simulink model "ofdm_13"  (Simulink 7.4)
settings: Solver=FixedStepDiscrete  SolverMode=SingleTasking  StartTime=0.0  StopTime=inf  MaxStep=1/(100*40e6)  RelTol=1e-3
PreLoadFcn:
  | Fsymbol              = .5e6;         % Symbol rate
  | D=8;  % decimation / interpolation
  | Bits_per_Symbol = 2;
  | Fbit  = Bits_per_Symbol*Fsymbol;
  | 
  | FFT_Size  = 64;
  | Cyclic        = 16;
  | Pilots         = 16;
  | Pilot_Level = 8;
  | Zero_Pad  = 3;
  | QAM_Level = 6;
  | 
  | OFDM_Frame =  FFT_Size+Cyclic;
  | Symbols_per_Frame = FFT_Size-Pilots-Zero_Pad;
  | 
  | Bits_per_Frame = Bits_per_Symbol*Symbols_per_Frame;
  | 
  | F_nco = Fsymbol*D*OFDM_Frame/(Symbols_per_Frame);
  | nco_nominal=2/D;
  | 
  | 
  | Fdelay = 8;  % rrc filter delay
  | Alpha = .25;  % excess BW
  | rrc_coef=rcosine(1,D,'fir/sqrt',Alpha,Fdelay);
  | rrc_coef=rrc_coef/sum(rrc_coef);
  | 
  | 
  | % coefficents for Farrow filter
  | b3 = [1/6 -1/2  1/2 -1/6];
  | b2 = [1/2 -1    1/2  0];
  | b1 = [1/3  1/2 -1    1/6];
  | b0 = [0    1    0    0];
StartFcn:
  | tic
StopFcn:
  | trun=toc
values from neighbouring files (symbols this model uses):
  Fs = 1    [16 qam.m]    (also in G.m = input('Enter sampling frequency='))
  j = imread('lena.jpg')    [ansk3.m]    (also in cosine_filter.m = 2; imag1.m)
  N = [N1;N2;N1_;N2_]    [FFT_OFDM_MIMO.m]    (also in MRCplot.m = 1000000; SDplot.m = 1000000; ansk2.m = 10; ansk3.m = 10)
undefined symbols (not defined in the file or in its folder): dBW, dfilt, Hz, magnitude, sided, Ts, Two
libraries: simulink x25, dspobslib x22, dspsigops x13, dspbuff3 x5, dspsnks4 x4, dspxfrm3 x4, dspstat3 x4, commsink2 x3, commchan3 x2, dsparch4 x2, commrandsrc2 x2, commdigbbndam3 x2
(part 2 of 2)

== system ofdm_13/OFDM Transmitter with Variable Symbol Timing and Carrier Frequency Error/Discrete-Time NCO ==
  note: initial condx=Ph
  note: VCO Sensitivity
  note: Center Freq
  note: Phase Accumulator
      | Modulus
  note: Amplitude
  in_1 : Inport  OutDataType=sfix(16)  OutScaling=2^0
  Discrete Constant1 : dspobslib/DSP Constant  SystemSampleTime=-1  Value=Fc*pi2*ts  SampleMode=Discrete  discreteOutput=Sample-based (interpret vectors as 1-D)  continuousOutput=Sample-based  sampTime=ts  framePeriod=ts  dataType=Inherit via back propagation  isSigned=on  wordLen=16  udDataType=sfix(16)  fracBitsMode=Best precision  numFracBits=15  InterpretAs1D=on  Ts=ts  FramebasedOutput=off
      settings: additionalParams=on
  Discrete Constant2 : dspobslib/DSP Constant  SystemSampleTime=-1  Value=pi2  SampleMode=Discrete  discreteOutput=Sample-based (interpret vectors as 1-D)  continuousOutput=Sample-based  sampTime=ts  framePeriod=ts  dataType=Inherit via back propagation  isSigned=on  wordLen=16  udDataType=sfix(16)  fracBitsMode=Best precision  numFracBits=15  InterpretAs1D=on  Ts=ts  FramebasedOutput=off
      settings: additionalParams=on
  Math Function : Math  Operator=mod  OutDataType=sfix(16)  OutScaling=2^0  SaturateOnIntegerOverflow=on
  Real-Imag to Complex : RealImagToComplex
  Sensitivity : Gain  Gain=Kc*pi2*ts  ParameterDataType=sfix(16)  ParameterScaling=2^0  OutDataType=sfix(16)  OutScaling=2^0  SaturateOnIntegerOverflow=on  OutDataTypeStr=Inherit: Same as input  ParamDataTypeStr=Inherit: Same as input
  Sensitivity2 : Gain  Gain=Ac  ParameterDataType=sfix(16)  ParameterScaling=2^0  OutDataType=sfix(16)  OutScaling=2^0  SaturateOnIntegerOverflow=on  OutDataTypeStr=Inherit: Same as input  ParamDataTypeStr=Inherit: Same as input
  Sum1 : Sum  Inputs=+++  OutDataType=sfix(16)  OutScaling=2^0  SaturateOnIntegerOverflow=on  InputSameDT=on  OutDataTypeStr=Inherit: Same as first input
  Trigonometric Function : Trigonometry  Operator=cos
  Trigonometric Function1 : Trigonometry
  Unit Delay : UnitDelay  X0=Ph  SampleTime=ts
  out_1 : Outport  OutDataType=sfix(16)  OutScaling=2^0  InitialOutput=0
  wires:
  Real-Imag to Complex/1 -> Sensitivity2/1
  Trigonometric Function1/1 -> Real-Imag to Complex/2
  Discrete Constant2/1 -> Math Function/2
  Sum1/1 -> Math Function/1
  Math Function/1 -> Unit Delay/1
  in_1/1 -> Sensitivity/1
  Sensitivity/1 -> Sum1/1
  Unit Delay/1 -> Trigonometric Function/1, Trigonometric Function1/1, Sum1/3
  Trigonometric Function/1 -> Real-Imag to Complex/1
  Sensitivity2/1 -> out_1/1
  Discrete Constant1/1 -> Sum1/2

== system ofdm_13/OFDM Transmitter with Variable Symbol Timing and Carrier Frequency Error/Farrow Variable Delay ==
  Xin : Inport  OutDataType=sfix(16)  OutScaling=2^0
  Mu : Inport  Port=2  OutDataType=sfix(16)  OutScaling=2^0
  Filter State : Subsystem
  MADS : Subsystem
  Yout : Outport  OutDataType=sfix(16)  OutScaling=2^0
  wires:
  Filter State/1(Out1) -> MADS/1(In1)
  Xin/1 -> Filter State/1(In1)
  Mu/1 -> MADS/2(mu)
  MADS/1(Yout) -> Yout/1

== system ofdm_13/OFDM Transmitter with Variable Symbol Timing and Carrier Frequency Error/OFDM Symbol Gen ==
  note: Output Samples Serially
  note: Note: Ouptut is SET TO ZERO
      | when not enabled.
      | This effecitvly inserts ZEROS in the stream
      | for proper interpolation.
  Enable : EnablePort
  Divide by  OFDM_Frame length : Subsystem  TreatAsAtomicUnit=on  mask(Pulse Divider){div=OFDM_Frame, ph=0}
      mask prompts: div "Modulo:"; ph "Initial Phase Delay (cycles):"
  OFDM Generator : Subsystem
  Selector : Selector  InputPortWidth=80  IndexOptions=Index vector (port)  Indices=[1 3]  OutputSizes=1
  Serial Samples Out : Outport  OutDataType=sfix(16)  OutScaling=2^0  OutputWhenDisabled=reset  InitialOutput=0+j*eps
  wires:
  OFDM Generator/1(Out1) -> Selector/1
  Divide by  OFDM_Frame length/1(Enable) -> OFDM Generator/Enable
  Selector/1 -> Serial Samples Out/1
  Divide by  OFDM_Frame length/2(Count) -> Selector/2

== system ofdm_13/OFDM Transmitter with Variable Symbol Timing and Carrier Frequency Error/Timing Control Unit1 ==
  note: Numerically Controlled Oscillator
  Control In : Inport  OutDataType=sfix(16)  OutScaling=2^0
  Delay2 : dspsigops/Delay  dly_unit=Samples  delay=1  ic_detail=on  dif_ic_for_ch=off  dif_ic_for_dly=off  ic=0  reset_popup=None
  Discrete Constant1 : dspobslib/DSP Constant  SystemSampleTime=-1  Value=1  SampleMode=Discrete  discreteOutput=Sample-based (interpret vectors as 1-D)  continuousOutput=Sample-based  sampTime=inf  framePeriod=inf  dataType=Inherit via back propagation  isSigned=on  wordLen=16  udDataType=sfix(16)  fracBitsMode=Best precision  numFracBits=15  InterpretAs1D=on  Ts=inf  FramebasedOutput=off
      settings: additionalParams=on
  Math Function : Math  Operator=mod  OutDataType=sfix(16)  OutScaling=2^0  SaturateOnIntegerOverflow=on
  Relational Operator1 : RelationalOperator  Operator=~=  LogicOutDataTypeMode=boolean  LogicDataType=double(64)  OutDataTypeStr=boolean
  S&H 1 : Subsystem  TreatAsAtomicUnit=on
  Scaling1 : Subsystem
  Sum2 : Sum  Inputs=-+  OutDataType=sfix(16)  OutScaling=2^0  SaturateOnIntegerOverflow=on  InputSameDT=on  OutDataTypeStr=Inherit: Same as first input
  Clock Out : Outport  OutDataType=sfix(16)  OutScaling=2^0
  Delay Control : Outport  Port=2  OutDataType=sfix(16)  OutScaling=2^0
  wires:
  Scaling1/1(Out1) -> Delay Control/1
  S&H 1/1(Out1) -> Scaling1/1(In1)
  Delay2/1 -> Math Function/1, Relational Operator1/1
  Discrete Constant1/1 -> Math Function/2
  Sum2/1 -> Delay2/1
  Math Function/1 -> Relational Operator1/2, S&H 1/1(In1), Sum2/2
  Relational Operator1/1 -> Clock Out/1, S&H 1/Enable
  Control In/1 -> Sum2/1, Scaling1/2(In2)

== system ofdm_13/Serial to Parallel and Frame Offset Est/Cyclic Prefix Correlation for Frame  Boundary Estimation ==
  note: http://citeseer.ist.psu.edu/cache/papers/cs/27222/http:zSzzSzwww.sm.luth.sezSzcseezSzspzSzresearchzSzconferencezSzbsb96c.pdf/on-synchronization-in-ofdm.pdf
  note: Google " On Synchronization in OFDM Systems Using the Cyclic Prefix "
  Strobe : Inport
  Serial : Inport  Port=2
  Estimators : Subsystem
  Find max : Subsystem
  Terminator : Terminator
  buffer one frame worth : dspbuff3/Delay Line  siz=OFDM_Frame  ic=0  directfeed=on  enable_output=off  hold_output=off
  Offset in Samples : Outport
  wires:
  Estimators/1(Delay Est Data) -> buffer one frame worth/1
  buffer one frame worth/1 -> Find max/1(In1)
  Estimators/2(Freq Error Est) -> Terminator/1
  Strobe/1 -> Find max/Enable
  Serial/1 -> Estimators/1(In1)
  Find max/1(Frame Offset Est) -> Offset in Samples/1

== system ofdm_13/Timing Control Unit/Compute % Error from Nominal value ==
  In : Inport
  Add : Sum  Inputs=+-  OutDataType=sfix(16)  OutScaling=2^-10
  Discrete Constant3 : dspobslib/DSP Constant  SystemSampleTime=-1  Value=1  SampleMode=Discrete  discreteOutput=Sample-based (interpret vectors as 1-D)  continuousOutput=Sample-based  sampTime=2/F_nco  framePeriod=2/F_nco  dataType=Inherit via back propagation  isSigned=on  wordLen=16  udDataType=sfix(16)  fracBitsMode=Best precision  numFracBits=15  InterpretAs1D=on  Ts=2/F_nco  FramebasedOutput=off
      settings: additionalParams=on
  Gain : Gain  Gain=1/nco_nominal  ParameterDataType=sfix(16)  ParameterScaling=2^0  OutDataType=sfix(16)  OutScaling=2^0
  Gain1 : Gain  Gain=100  ParameterDataType=sfix(16)  ParameterScaling=2^0  OutDataType=sfix(16)  OutScaling=2^0
  Out : Outport
  wires:
  Gain1/1 -> Out/1
  In/1 -> Gain/1
  Discrete Constant3/1 -> Add/2
  Add/1 -> Gain1/1
  Gain/1 -> Add/1

== system ofdm_13/Timing Control Unit/Sample & Scale ==
  In1 : Inport  OutDataType=sfix(16)  OutScaling=2^0
  In2 : Inport  Port=2  OutDataType=sfix(16)  OutScaling=2^0
  Enable : EnablePort
  Discrete Constant2 : dspobslib/DSP Constant  SystemSampleTime=-1  Value=-1  SampleMode=Discrete  discreteOutput=Sample-based (interpret vectors as 1-D)  continuousOutput=Sample-based  sampTime=inf  framePeriod=inf  dataType=Inherit via back propagation  isSigned=on  wordLen=16  udDataType=sfix(16)  fracBitsMode=Best precision  numFracBits=15  InterpretAs1D=on  Ts=inf  FramebasedOutput=off
      settings: additionalParams=on
  Product : Product  Inputs=*/  OutDataType=sfix(16)  OutScaling=2^0  RndMeth=Zero
  Sum1 : Sum  OutDataType=sfix(16)  OutScaling=2^0  SaturateOnIntegerOverflow=on  InputSameDT=on  OutDataTypeStr=Inherit: Same as first input
  Out1 : Outport  OutDataType=sfix(16)  OutScaling=2^0
  wires:
  Product/1 -> Sum1/1
  Discrete Constant2/1 -> Sum1/2
  In1/1 -> Product/1
  Sum1/1 -> Out1/1
  In2/1 -> Product/2

== system ofdm_13/OFDM Rx/OFDM Receiver/Remove pilots ==
  note: Get Data Sans
      | 3 Zero Channels
  "  " : Inport  OutDataType=sfix(16)  OutScaling=2^0
  Selector : Selector  InputPortWidth=64  IndexOptions=Index vector (dialog)  Indices="[   4:6   8:10  12:14  16:18  20:22  24:26  28:30   32:34  36:38    40:42     44:46   48:50  52:54  56:58   60:62   ]"  OutputSizes=1
  Selector1 : Selector  InputPortWidth=64  IndexOptions=Index vector (dialog)  Indices=[0 1 2 3 4 5 6 7 8 9 10 11 12 13 14 15 ]*4 +3  OutputSizes=1
  Data : Outport  OutDataType=sfix(16)  OutScaling=2^0
  Pilots : Outport  Port=2  OutDataType=sfix(16)  OutScaling=2^0
  wires:
  "  "/1 -> Selector/1, Selector1/1
  Selector/1 -> Data/1
  Selector1/1 -> Pilots/1

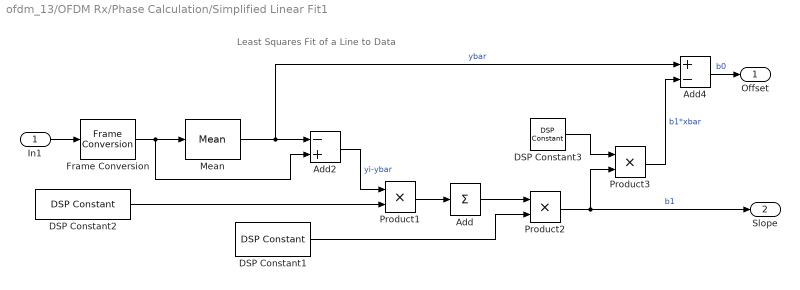
== system ofdm_13/OFDM Rx/Phase Calculation/Simplified Linear Fit1 ==
  note: Least Squares Fit of a Line to Data
  In1 : Inport
  Add : Sum  Inputs=+  OutDataType=sfix(16)  OutScaling=2^-10
  Add2 : Sum  Inputs=-+  OutDataType=sfix(16)  OutScaling=2^-10
  Add4 : Sum  Inputs=+-  OutDataType=sfix(16)  OutScaling=2^-10
  DSP Constant1 : dspobslib/DSP Constant  SystemSampleTime=-1  Value=1/14630  SampleMode=Discrete  discreteOutput=Sample-based  continuousOutput=Sample-based  sampTime=inf  framePeriod=N*Ts  dataType=Inherit from 'Constant value'  isSigned=on  wordLen=16  udDataType=sfix(16)  fracBitsMode=Best precision  numFracBits=15  InterpretAs1D=-inf  Ts=-inf  FramebasedOutput=-inf
  DSP Constant2 : dspobslib/DSP Constant  SystemSampleTime=-1  Value=[-27.5:27.5]'  SampleMode=Discrete  discreteOutput=Sample-based  continuousOutput=Sample-based  sampTime=inf  framePeriod=N*Ts  dataType=Inherit from 'Constant value'  isSigned=on  wordLen=16  udDataType=sfix(16)  fracBitsMode=Best precision  numFracBits=15  InterpretAs1D=-inf  Ts=-inf  FramebasedOutput=-inf
  DSP Constant3 : dspobslib/DSP Constant  SystemSampleTime=-1  Value=-.5  SampleMode=Discrete  discreteOutput=Sample-based  continuousOutput=Sample-based  sampTime=inf  framePeriod=N*Ts  dataType=Inherit from 'Constant value'  isSigned=on  wordLen=16  udDataType=sfix(16)  fracBitsMode=Best precision  numFracBits=15  InterpretAs1D=-inf  Ts=-inf  FramebasedOutput=-inf
  Frame Conversion : FrameConversion  OutFrame=Sample-based
  Mean : dspstat3/Mean  DialogController=dspDDGCreate  DialogControllerArgs=DataTag9  run=off  reset_popup=None  directionMode=Each column  dimension=1  treatSBRowAsCol=on  roiEnable=off  roiType=Rectangles  roiPortion=Entire ROI  roiOutput=Individual statistics for each ROI  roiFlag=off  outputDataTypeStr=Inherit: Same as accumulator  outputLastDataTypeStr=Inherit: Same as accumulator  outputMin=[]  outputMax=[]  roundingMode=Floor  overflowMode=off
  Product1 : Product  OutDataType=sfix(16)  OutScaling=2^0  RndMeth=Zero
  Product2 : Product  Inputs=**  OutDataType=sfix(16)  OutScaling=2^0  RndMeth=Zero
  Product3 : Product  Inputs=**  OutDataType=sfix(16)  OutScaling=2^0  RndMeth=Zero
  Offset : Outport
  Slope : Outport  Port=2
  wires:
  Frame Conversion/1 -> Mean/1, Add2/2
  DSP Constant3/1 -> Product3/1
  DSP Constant2/1 -> Product1/2
  DSP Constant1/1 -> Product2/2
  Mean/1 -> Add2/1, Add4/1  "ybar"
  Add2/1 -> Product1/1  "yi-ybar"
  Product1/1 -> Add/1
  Add/1 -> Product2/1
  Product2/1 -> Product3/2, Slope/1  "b1"
  Product3/1 -> Add4/2  "b1*xbar"
  In1/1 -> Frame Conversion/1
  Add4/1 -> Offset/1  "b0"

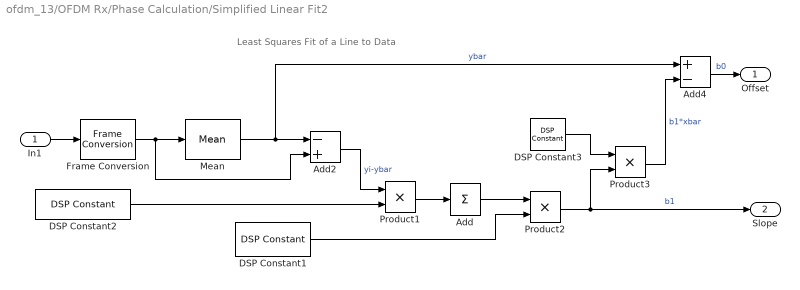
== system ofdm_13/OFDM Rx/Phase Calculation/Simplified Linear Fit2 ==
  note: Least Squares Fit of a Line to Data
  In1 : Inport
  Add : Sum  Inputs=+  OutDataType=sfix(16)  OutScaling=2^-10
  Add2 : Sum  Inputs=-+  OutDataType=sfix(16)  OutScaling=2^-10
  Add4 : Sum  Inputs=+-  OutDataType=sfix(16)  OutScaling=2^-10
  DSP Constant1 : dspobslib/DSP Constant  SystemSampleTime=-1  Value=1/14630  SampleMode=Discrete  discreteOutput=Sample-based  continuousOutput=Sample-based  sampTime=inf  framePeriod=N*Ts  dataType=Inherit from 'Constant value'  isSigned=on  wordLen=16  udDataType=sfix(16)  fracBitsMode=Best precision  numFracBits=15  InterpretAs1D=-inf  Ts=-inf  FramebasedOutput=-inf
  DSP Constant2 : dspobslib/DSP Constant  SystemSampleTime=-1  Value=[-27.5:27.5]'  SampleMode=Discrete  discreteOutput=Sample-based  continuousOutput=Sample-based  sampTime=inf  framePeriod=N*Ts  dataType=Inherit from 'Constant value'  isSigned=on  wordLen=16  udDataType=sfix(16)  fracBitsMode=Best precision  numFracBits=15  InterpretAs1D=-inf  Ts=-inf  FramebasedOutput=-inf
  DSP Constant3 : dspobslib/DSP Constant  SystemSampleTime=-1  Value=-.5  SampleMode=Discrete  discreteOutput=Sample-based  continuousOutput=Sample-based  sampTime=inf  framePeriod=N*Ts  dataType=Inherit from 'Constant value'  isSigned=on  wordLen=16  udDataType=sfix(16)  fracBitsMode=Best precision  numFracBits=15  InterpretAs1D=-inf  Ts=-inf  FramebasedOutput=-inf
  Frame Conversion : FrameConversion  OutFrame=Sample-based
  Mean : dspstat3/Mean  DialogController=dspDDGCreate  DialogControllerArgs=DataTag10  run=off  reset_popup=None  directionMode=Each column  dimension=1  treatSBRowAsCol=on  roiEnable=off  roiType=Rectangles  roiPortion=Entire ROI  roiOutput=Individual statistics for each ROI  roiFlag=off  outputDataTypeStr=Inherit: Same as accumulator  outputLastDataTypeStr=Inherit: Same as accumulator  outputMin=[]  outputMax=[]  roundingMode=Floor  overflowMode=off
  Product1 : Product  OutDataType=sfix(16)  OutScaling=2^0  RndMeth=Zero
  Product2 : Product  Inputs=**  OutDataType=sfix(16)  OutScaling=2^0  RndMeth=Zero
  Product3 : Product  Inputs=**  OutDataType=sfix(16)  OutScaling=2^0  RndMeth=Zero
  Offset : Outport
  Slope : Outport  Port=2
  wires:
  Add4/1 -> Offset/1  "b0"
  In1/1 -> Frame Conversion/1
  Product3/1 -> Add4/2  "b1*xbar"
  Product2/1 -> Slope/1, Product3/2  "b1"
  Add/1 -> Product2/1
  Product1/1 -> Add/1
  Add2/1 -> Product1/1  "yi-ybar"
  Mean/1 -> Add4/1, Add2/1  "ybar"
  DSP Constant1/1 -> Product2/2
  DSP Constant2/1 -> Product1/2
  DSP Constant3/1 -> Product3/1
  Frame Conversion/1 -> Add2/2, Mean/1

== system ofdm_13/OFDM Transmitter with Variable Symbol Timing and Carrier Frequency Error/Farrow Variable Delay/Filter State ==
  In1 : Inport  OutDataType=sfix(16)  OutScaling=2^0
  Delay : dspsigops/Delay  dly_unit=Samples  delay=1  ic_detail=off  dif_ic_for_ch=off  dif_ic_for_dly=off  ic=0  reset_popup=None
  Delay1 : dspsigops/Delay  dly_unit=Samples  delay=1  ic_detail=off  dif_ic_for_ch=off  dif_ic_for_dly=off  ic=0  reset_popup=None
  Delay2 : dspsigops/Delay  dly_unit=Samples  delay=1  ic_detail=off  dif_ic_for_ch=off  dif_ic_for_dly=off  ic=0  reset_popup=None
  Mux : Mux
  Out1 : Outport  OutDataType=sfix(16)  OutScaling=2^0
  wires:
  In1/1 -> Delay/1, Mux/1
  Delay/1 -> Mux/2, Delay1/1
  Delay1/1 -> Mux/3, Delay2/1
  Delay2/1 -> Mux/4
  Mux/1 -> Out1/1

== system ofdm_13/OFDM Transmitter with Variable Symbol Timing and Carrier Frequency Error/Farrow Variable Delay/MADS ==
  note: Horner's Rule
  note: Filter Coefficients from Chris Dick Xilinx,
      | or H. Meyer pp 520 (9-33) Digital Communications Receivers
  In1 : Inport  OutDataType=sfix(16)  OutScaling=2^0
  mu : Inport  Port=2  OutDataType=sfix(16)  OutScaling=2^0
  Demux : Demux
  Filter coefficients : Gain  Gain="[b3;b2;b1;b0]   % filter coefficients"  Multiplication=Matrix(K*u)  ParameterDataType=sfix(16)  ParameterScaling=2^0  OutDataType=sfix(16)  OutScaling=2^0  SaturateOnIntegerOverflow=on  OutDataTypeStr=Inherit: Same as input  ParamDataTypeStr=Inherit: Same as input
  P1 : Product  OutDataType=sfix(16)  OutScaling=2^0  SaturateOnIntegerOverflow=on  OutDataTypeStr=Inherit: Same as first input
  P2 : Product  OutDataType=sfix(16)  OutScaling=2^0  SaturateOnIntegerOverflow=on  OutDataTypeStr=Inherit: Same as first input
  P3 : Product  OutDataType=sfix(16)  OutScaling=2^0  SaturateOnIntegerOverflow=on  OutDataTypeStr=Inherit: Same as first input
  Sum1 : Sum  Inputs=|++  OutDataType=sfix(16)  OutScaling=2^0  SaturateOnIntegerOverflow=on
  Sum2 : Sum  Inputs=|++  OutDataType=sfix(16)  OutScaling=2^0  SaturateOnIntegerOverflow=on
  Sum3 : Sum  Inputs=|++  OutDataType=sfix(16)  OutScaling=2^0  SaturateOnIntegerOverflow=on
  Yout : Outport  OutDataType=sfix(16)  OutScaling=2^0
  wires:
  P3/1 -> Sum3/1
  P2/1 -> Sum2/1
  Filter coefficients/1 -> Demux/1
  In1/1 -> Filter coefficients/1
  mu/1 -> P3/1, P2/1, P1/1
  Demux/1 -> P1/2
  Sum1/1 -> P2/2
  Sum2/1 -> P3/2
  Demux/2 -> Sum1/2
  P1/1 -> Sum1/1
  Demux/3 -> Sum2/2
  Demux/4 -> Sum3/2
  Sum3/1 -> Yout/1

== system ofdm_13/OFDM Transmitter with Variable Symbol Timing and Carrier Frequency Error/OFDM Symbol Gen/Divide by  OFDM_Frame length ==
  Constant1 : Constant  Value=div  OutDataType=sfix(16)  OutScaling=2^0
  Constant2 : Constant  OutDataType=sfix(16)  OutScaling=2^0
  Fcn4 : Fcn  Expr=u<1
  Math Function : Math  Operator=mod  OutDataType=sfix(16)  OutScaling=2^0  SaturateOnIntegerOverflow=on
  Sum : Sum  Inputs=|++  OutDataType=sfix(16)  OutScaling=2^0  SaturateOnIntegerOverflow=on  InputSameDT=on  OutDataTypeStr=Inherit: Same as first input
  Unit Delay : UnitDelay  X0=div-ph  SampleTime=-1
  Enable : Outport  OutDataType=sfix(16)  OutScaling=2^0
  Count : Outport  Port=2  OutDataType=sfix(16)  OutScaling=2^0
  wires:
  Sum/1 -> Unit Delay/1, Count/1
  Constant2/1 -> Sum/1
  Unit Delay/1 -> Math Function/1
  Math Function/1 -> Sum/2, Fcn4/1
  Constant1/1 -> Math Function/2
  Fcn4/1 -> Enable/1

== system ofdm_13/OFDM Transmitter with Variable Symbol Timing and Carrier Frequency Error/OFDM Symbol Gen/OFDM Generator ==
  note: set data signal level
  Enable : EnablePort
  Bernoulli Random Binary Generator : commrandsrc2/Bernoulli Binary Generator  DialogController=commDDGCreate  DialogControllerArgs=DataTag12  SystemSampleTime=-1  P=0.5  seed=123  Ts=-1  frameBased=on  sampPerFrame=Bits_per_Frame  orient=off  outDataType=double
  Frame Conversion : FrameConversion  OutFrame=Sample-based
  Gain : Gain  Gain=D  ParameterDataType=sfix(16)  ParameterScaling=2^0  OutDataType=sfix(16)  OutScaling=2^0
  Gain1 : Gain  Gain=QAM_Level  ParameterDataType=sfix(16)  ParameterScaling=2^0  OutDataType=sfix(16)  OutScaling=2^0  SaturateOnIntegerOverflow=on  OutDataTypeStr=Inherit: Same as input  ParamDataTypeStr=Inherit: Same as input
  OFDM Transmitter1 : Subsystem
      mask Display: disp('OFDM\nTransmitter')
  Rectangular QAM Modulator Baseband1 : commdigbbndam3/Rectangular QAM Modulator Baseband  DialogController=commDDGCreate  DialogControllerArgs=DataTag14  M=4  InType=Bit  Enc=Binary  Mapping=[0:15]  PowType=Min. distance between symbols  MinDist=2  AvgPow=1  PeakPow=1  Ph=0  outDtype=double  outWordLen=16  outUDDataType=sfix(16)  outFracLenMode=Best precision  outFracLen=15
  Out1 : Outport  OutDataType=sfix(16)  OutScaling=2^0
  wires:
  Bernoulli Random Binary Generator/1 -> Rectangular QAM Modulator Baseband1/1
  OFDM Transmitter1/1(Out) -> Gain/1
  Rectangular QAM Modulator Baseband1/1 -> Gain1/1
  Gain/1 -> Frame Conversion/1
  Gain1/1 -> OFDM Transmitter1/1(In)
  Frame Conversion/1 -> Out1/1

== system ofdm_13/OFDM Transmitter with Variable Symbol Timing and Carrier Frequency Error/Timing Control Unit1/S&H 1 ==
  In1 : Inport  OutDataType=sfix(16)  OutScaling=2^0
  Enable : EnablePort
  Out1 : Outport  OutDataType=sfix(16)  OutScaling=2^0
  wires:
  In1/1 -> Out1/1

== system ofdm_13/OFDM Transmitter with Variable Symbol Timing and Carrier Frequency Error/Timing Control Unit1/Scaling1 ==
  note: This Division can be eliminated
      | and replaced by a mpy by constant
      | for small variations (< 1%)
      | about an operating point.
  In1 : Inport  OutDataType=sfix(16)  OutScaling=2^0
  In2 : Inport  Port=2  OutDataType=sfix(16)  OutScaling=2^0
  Add : Sum  Inputs=-+  OutDataType=sfix(16)  OutScaling=2^-10
  Constant : Constant  OutDataType=sfix(16)  OutScaling=2^0
  Divide : Product  Inputs=*/  OutDataType=sfix(16)  OutScaling=2^-10
  Out1 : Outport  OutDataType=sfix(16)  OutScaling=2^0
  wires:
  In2/1 -> Divide/2
  In1/1 -> Add/1
  Constant/1 -> Add/2
  Add/1 -> Divide/1
  Divide/1 -> Out1/1

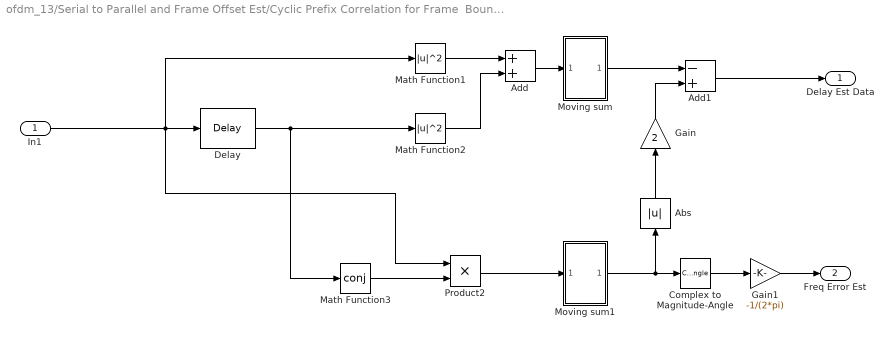
== system ofdm_13/Serial to Parallel and Frame Offset Est/Cyclic Prefix Correlation for Frame  Boundary Estimation/Estimators ==
  In1 : Inport  OutDataType=sfix(16)  OutScaling=2^0
  Abs : Abs
  Add : Sum  OutDataType=sfix(16)  OutScaling=2^-10
  Add1 : Sum  Inputs=-+  OutDataType=sfix(16)  OutScaling=2^-10
  Complex to Magnitude-Angle : ComplexToMagnitudeAngle  Output=Angle
  Delay : dspsigops/Delay  dly_unit=Samples  delay=FFT_Size  ic_detail=off  dif_ic_for_ch=off  dif_ic_for_dly=off  ic=0  reset_popup=None
  Gain : Gain  Gain=2  ParameterDataType=sfix(16)  ParameterScaling=2^0  OutDataType=sfix(16)  OutScaling=2^0
  Gain1 : Gain  Gain=-1/(2*pi)  ParameterDataType=sfix(16)  ParameterScaling=2^0  OutDataType=sfix(16)  OutScaling=2^0
  Math Function1 : Math  Operator=magnitude^2  OutDataType=sfix(16)  OutScaling=2^0  SaturateOnIntegerOverflow=on
  Math Function2 : Math  Operator=magnitude^2  OutDataType=sfix(16)  OutScaling=2^0  SaturateOnIntegerOverflow=on
  Math Function3 : Math  Operator=conj  OutDataType=sfix(16)  OutScaling=2^0  SaturateOnIntegerOverflow=on
  Moving sum : Subsystem
  Moving sum1 : Subsystem
  Product2 : Product  OutDataType=sfix(16)  OutScaling=2^0  RndMeth=Zero
  Delay Est Data : Outport  OutDataType=sfix(16)  OutScaling=2^0
  Freq Error Est : Outport  Port=2  OutDataType=sfix(16)  OutScaling=2^0
  wires:
  In1/1 -> Product2/1, Delay/1, Math Function1/1
  Gain1/1 -> Freq Error Est/1
  Complex to Magnitude-Angle/1 -> Gain1/1
  Math Function3/1 -> Product2/2
  Gain/1 -> Add1/2
  Abs/1 -> Gain/1
  Add1/1 -> Delay Est Data/1
  Moving sum/1(Out1) -> Add1/1
  Moving sum1/1(Out1) -> Complex to Magnitude-Angle/1, Abs/1
  Product2/1 -> Moving sum1/1(In1)
  Add/1 -> Moving sum/1(In1)
  Math Function2/1 -> Add/2
  Math Function1/1 -> Add/1
  Delay/1 -> Math Function3/1, Math Function2/1

== system ofdm_13/Serial to Parallel and Frame Offset Est/Cyclic Prefix Correlation for Frame  Boundary Estimation/Find max ==
  In1 : Inport
  Enable : EnablePort
  Add : Sum  Inputs=+-  OutDataType=sfix(16)  OutScaling=2^-10
  Constant : Constant  Value=OFDM_Frame/2  OutDataType=sfix(16)  OutScaling=2^0
  Frame Conversion : FrameConversion  OutFrame=Sample-based
  Maximum : dspstat3/Maximum  DialogController=dspDDGCreate  DialogControllerArgs=DataTag18  fcn=Index  reset=None  indexBase=One  operateOver=Each column  Dimension=1  colComp=on  operation=maximum  roiEnable=off  roiType=Rectangles  roiPortion=Entire ROI  roiOutput=Individual statistics for each ROI  roiFlag=off  accumDataTypeStr=Inherit: Same as product output  accumLastDataTypeStr=Inherit: Same as product output  roundingMode=Floor  overflowMode=off
  Moving sum : Subsystem
  reorder to center 0 point : Selector  InputPortWidth=80  IndexOptions=Index vector (dialog)  Indices=[(OFDM_Frame/2+1):80 1:OFDM_Frame/2]  OutputSizes=1
  Frame Offset Est : Outport  InitialOutput=0
  wires:
  In1/1 -> reorder to center 0 point/1
  Maximum/1 -> Frame Conversion/1
  reorder to center 0 point/1 -> Maximum/1
  Frame Conversion/1 -> Add/1
  Add/1 -> Moving sum/1(In1)
  Constant/1 -> Add/2
  Moving sum/1(Out1) -> Frame Offset Est/1

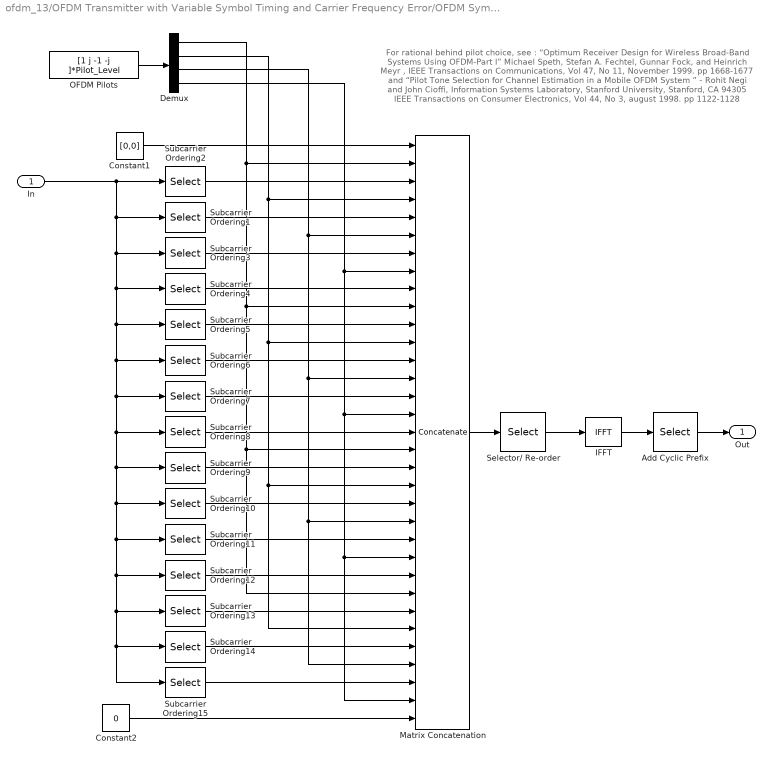
== system ofdm_13/OFDM Transmitter with Variable Symbol Timing and Carrier Frequency Error/OFDM Symbol Gen/OFDM Generator/OFDM Transmitter1 ==
  note: For rational behind pilot choice, see :
      | “Optimum Receiver Design for Wireless Broad-Band Systems Using OFDM-Part I”
      | Michael Speth, Stefan A. Fechtel, Gunnar Fock, and Heinrich Meyr ,
      |  IEEE Transactions on Communications, Vol 47, No 11, November 1999. pp 1668-1677
      | and
      | “Pilot Tone Selection for Channel Estimation in a Mobile OFDM System ” -
      |  Rohit Negi and John Cioffi, Information Systems Laboratory, Stanford University, Stanford, CA 94305
      | IEEE Transactions on Consumer Electronics, Vol 44, No 3, august 1998. pp 1122-1128
  In : Inport  OutDataType=sfix(16)  OutScaling=2^0
  Add Cyclic Prefix : Selector  InputPortWidth=64  IndexOptions=Index vector (dialog)  Indices=[49:64 1:64]  OutputSizes=1
  Constant1 : Constant  Value=[0,0]  OutDataType=sfix(16)  OutScaling=2^0
  Constant2 : Constant  Value=0  OutDataType=sfix(16)  OutScaling=2^0
  Demux : Demux
  IFFT : dspxfrm3/IFFT  DialogController=dspDDGCreate  DialogControllerArgs=DataTag13  CompMethod=Table lookup  TableOpt=HYBRID  TableOptActive=Speed  BitRevOrder=off  cs_in=off  SkipNorm=on  InheritFFTLength=on  FFTLength=64  mode=Complex  outSamplingMode=Frame based  roundingMode=Floor  overflowMode=off
  Matrix Concatenation : Concatenate  NumInputs=33  Mode=Multidimensional array
  OFDM Pilots : Constant  Value="[1 j -1 -j   ]*Pilot_Level"  OutDataType=sfix(16)  OutScaling=2^0
  Selector/ Re-order : Selector  InputPortWidth=64  IndexOptions=Index vector (dialog)  Indices=[33:64 1:32]  OutputSizes=1
  Subcarrier Ordering1 : Selector  InputPortWidth=Symbols_per_Frame  IndexOptions=Index vector (dialog)  Indices=4:6  OutputSizes=1
  Subcarrier Ordering10 : Selector  InputPortWidth=Symbols_per_Frame  IndexOptions=Index vector (dialog)  Indices=28:30  OutputSizes=1
  Subcarrier Ordering11 : Selector  InputPortWidth=Symbols_per_Frame  IndexOptions=Index vector (dialog)  Indices=31:33  OutputSizes=1
  Subcarrier Ordering12 : Selector  InputPortWidth=Symbols_per_Frame  IndexOptions=Index vector (dialog)  Indices=34:36  OutputSizes=1
  Subcarrier Ordering13 : Selector  InputPortWidth=Symbols_per_Frame  IndexOptions=Index vector (dialog)  Indices=37:39  OutputSizes=1
  Subcarrier Ordering14 : Selector  InputPortWidth=Symbols_per_Frame  IndexOptions=Index vector (dialog)  Indices=40:42  OutputSizes=1
  Subcarrier Ordering15 : Selector  InputPortWidth=Symbols_per_Frame  IndexOptions=Index vector (dialog)  Indices=43:45  OutputSizes=1
  Subcarrier Ordering2 : Selector  InputPortWidth=Symbols_per_Frame  IndexOptions=Index vector (dialog)  Indices=1:3  OutputSizes=1
  Subcarrier Ordering3 : Selector  InputPortWidth=Symbols_per_Frame  IndexOptions=Index vector (dialog)  Indices=7:9  OutputSizes=1
  Subcarrier Ordering4 : Selector  InputPortWidth=Symbols_per_Frame  IndexOptions=Index vector (dialog)  Indices=10:12  OutputSizes=1
  Subcarrier Ordering5 : Selector  InputPortWidth=Symbols_per_Frame  IndexOptions=Index vector (dialog)  Indices=13:15  OutputSizes=1
  Subcarrier Ordering6 : Selector  InputPortWidth=Symbols_per_Frame  IndexOptions=Index vector (dialog)  Indices=16:18  OutputSizes=1
  Subcarrier Ordering7 : Selector  InputPortWidth=Symbols_per_Frame  IndexOptions=Index vector (dialog)  Indices=19:21  OutputSizes=1
  Subcarrier Ordering8 : Selector  InputPortWidth=Symbols_per_Frame  IndexOptions=Index vector (dialog)  Indices=22:24  OutputSizes=1
  Subcarrier Ordering9 : Selector  InputPortWidth=Symbols_per_Frame  IndexOptions=Index vector (dialog)  Indices=25:27  OutputSizes=1
  Out : Outport  OutDataType=sfix(16)  OutScaling=2^0
  wires:
  In/1 -> Subcarrier Ordering14/1, Subcarrier Ordering15/1, Subcarrier Ordering13/1, Subcarrier Ordering12/1, Subcarrier Ordering11/1, Subcarrier Ordering10/1, Subcarrier Ordering9/1, Subcarrier Ordering8/1, Subcarrier Ordering7/1, Subcarrier Ordering6/1, Subcarrier Ordering5/1, Subcarrier Ordering4/1, Subcarrier Ordering3/1, Subcarrier Ordering1/1, Subcarrier Ordering2/1
  IFFT/1 -> Add Cyclic Prefix/1
  Matrix Concatenation/1 -> Selector/ Re-order/1
  Selector/ Re-order/1 -> IFFT/1
  Subcarrier Ordering2/1 -> Matrix Concatenation/3
  Subcarrier Ordering1/1 -> Matrix Concatenation/5
  Subcarrier Ordering3/1 -> Matrix Concatenation/7
  Subcarrier Ordering4/1 -> Matrix Concatenation/9
  Subcarrier Ordering5/1 -> Matrix Concatenation/11
  Subcarrier Ordering6/1 -> Matrix Concatenation/13
  Subcarrier Ordering7/1 -> Matrix Concatenation/15
  Subcarrier Ordering8/1 -> Matrix Concatenation/17
  Subcarrier Ordering9/1 -> Matrix Concatenation/19
  Subcarrier Ordering10/1 -> Matrix Concatenation/21
  Subcarrier Ordering11/1 -> Matrix Concatenation/23
  Subcarrier Ordering12/1 -> Matrix Concatenation/25
  Subcarrier Ordering13/1 -> Matrix Concatenation/27
  Subcarrier Ordering14/1 -> Matrix Concatenation/29
  Subcarrier Ordering15/1 -> Matrix Concatenation/31
  Add Cyclic Prefix/1 -> Out/1
  Constant1/1 -> Matrix Concatenation/1
  Constant2/1 -> Matrix Concatenation/33
  Demux/2 -> Matrix Concatenation/4, Matrix Concatenation/12, Matrix Concatenation/20, Matrix Concatenation/28
  Demux/3 -> Matrix Concatenation/6, Matrix Concatenation/14, Matrix Concatenation/22, Matrix Concatenation/30
  Demux/4 -> Matrix Concatenation/8, Matrix Concatenation/16, Matrix Concatenation/24, Matrix Concatenation/32
  OFDM Pilots/1 -> Demux/1
  Demux/1 -> Matrix Concatenation/26, Matrix Concatenation/18, Matrix Concatenation/10, Matrix Concatenation/2

== system ofdm_13/Serial to Parallel and Frame Offset Est/Cyclic Prefix Correlation for Frame  Boundary Estimation/Estimators/Moving sum ==
  In1 : Inport  OutDataType=sfix(16)  OutScaling=2^0
  Gain : Gain  Gain=1/Cyclic  ParameterDataType=sfix(16)  ParameterScaling=2^0  OutDataType=sfix(16)  OutScaling=2^0  SaturateOnIntegerOverflow=on  OutDataTypeStr=Inherit: Same as input  ParamDataTypeStr=Inherit: Same as input
  Integer Delay : simulink/Discrete/Integer Delay  vinit=0.0  samptime=-1  NumDelays=Cyclic
  Integer Delay1 : simulink/Discrete/Integer Delay  vinit=0.0  samptime=-1  NumDelays=1
  Sum2 : Sum  Inputs=|+-  OutDataType=sfix(16)  OutScaling=2^0
  Sum3 : Sum  Inputs=|++  OutDataType=sfix(16)  OutScaling=2^0
  Out1 : Outport  OutDataType=sfix(16)  OutScaling=2^0
  wires:
  Gain/1 -> Out1/1
  In1/1 -> Sum2/1, Integer Delay/1
  Sum2/1 -> Sum3/1
  Integer Delay1/1 -> Sum3/2
  Sum3/1 -> Gain/1, Integer Delay1/1
  Integer Delay/1 -> Sum2/2

== system ofdm_13/Serial to Parallel and Frame Offset Est/Cyclic Prefix Correlation for Frame  Boundary Estimation/Estimators/Moving sum1 ==
  In1 : Inport  OutDataType=sfix(16)  OutScaling=2^0
  Gain : Gain  Gain=1/Cyclic  ParameterDataType=sfix(16)  ParameterScaling=2^0  OutDataType=sfix(16)  OutScaling=2^0  SaturateOnIntegerOverflow=on  OutDataTypeStr=Inherit: Same as input  ParamDataTypeStr=Inherit: Same as input
  Integer Delay : simulink/Discrete/Integer Delay  vinit=0.0  samptime=-1  NumDelays=Cyclic
  Integer Delay1 : simulink/Discrete/Integer Delay  vinit=0.0  samptime=-1  NumDelays=1
  Sum2 : Sum  Inputs=|+-  OutDataType=sfix(16)  OutScaling=2^0
  Sum3 : Sum  Inputs=|++  OutDataType=sfix(16)  OutScaling=2^0
  Out1 : Outport  OutDataType=sfix(16)  OutScaling=2^0
  wires:
  Integer Delay/1 -> Sum2/2
  Sum3/1 -> Integer Delay1/1, Gain/1
  Integer Delay1/1 -> Sum3/2
  Sum2/1 -> Sum3/1
  In1/1 -> Integer Delay/1, Sum2/1
  Gain/1 -> Out1/1

== system ofdm_13/Serial to Parallel and Frame Offset Est/Cyclic Prefix Correlation for Frame  Boundary Estimation/Find max/Moving sum ==
  In1 : Inport  OutDataType=sfix(16)  OutScaling=2^0
  Gain : Gain  Gain=1/4  ParameterDataType=sfix(16)  ParameterScaling=2^0  OutDataType=sfix(16)  OutScaling=2^0  SaturateOnIntegerOverflow=on  OutDataTypeStr=Inherit: Same as input  ParamDataTypeStr=Inherit: Same as input
  Integer Delay : simulink/Discrete/Integer Delay  vinit=0.0  samptime=-1  NumDelays=4
  Integer Delay1 : simulink/Discrete/Integer Delay  vinit=0  samptime=-1  NumDelays=1
  Sum2 : Sum  Inputs=|+-  OutDataType=sfix(16)  OutScaling=2^0
  Sum3 : Sum  Inputs=|++  OutDataType=sfix(16)  OutScaling=2^0
  Out1 : Outport  OutDataType=sfix(16)  OutScaling=2^0
  wires:
  Integer Delay/1 -> Sum2/2
  Sum3/1 -> Integer Delay1/1, Gain/1
  Integer Delay1/1 -> Sum3/2
  Sum2/1 -> Sum3/1
  In1/1 -> Integer Delay/1, Sum2/1
  Gain/1 -> Out1/1
